simulink model "cc_main_multiple_points"  (R2016b)
settings: Solver=FixedStepAuto  StartTime=0.0  StopTime=inf  FixedStep=1e-3  RelTol=1e-3
values from neighbouring files (symbols this model uses):
  lx = 10    [multiple_points_platform_and_ball_characteristics.m]
  ly = 10    [multiple_points_platform_and_ball_characteristics.m]
libraries: MBDyn_collision_activator x3, MBDynCom x2
settings Model: Creator=matteo  LastModifiedBy=matteo

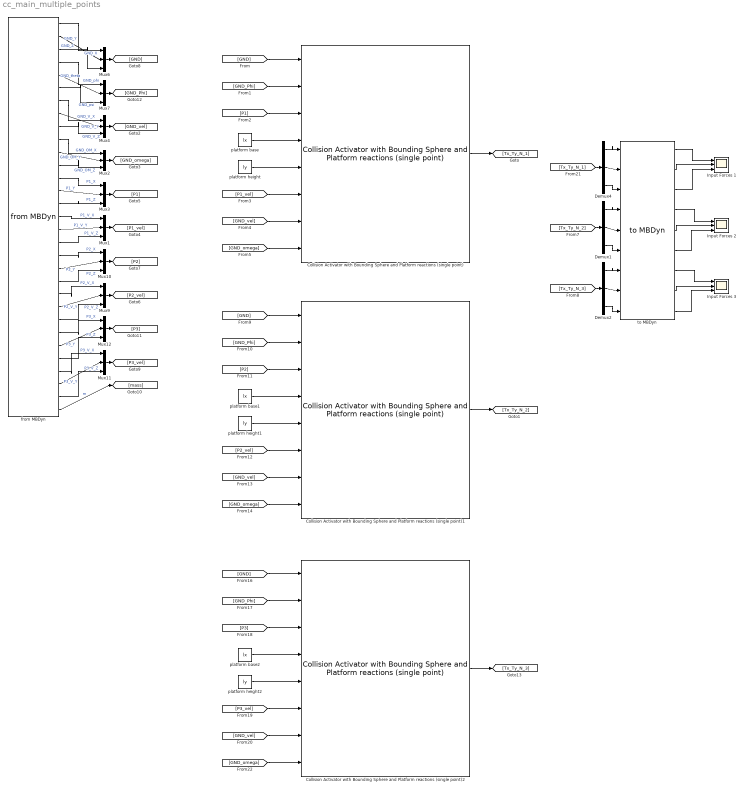
== system cc_main_multiple_points ==
  Collision Activator with Bounding Sphere and Platform reactions (single point) : MBDyn_collision_activator/Collision Activator with Bounding Sphere and Platform reactions (single point)  mult_factor=10  coulomb_friction_value=0  coefficient_viscous_friction=0.05  cosine_flag_threshold=3.9  local_distance_from_gnd_threshold=0  ground_stiffness=1e9  restitution_coeff=0.8  impact_speed_threshold=0.2  reaction_force_exponential=3  force_sign=-1  dissipation_coefficient_model=Flores
  Collision Activator with Bounding Sphere and Platform reactions (single point)1 : MBDyn_collision_activator/Collision Activator with Bounding Sphere and Platform reactions (single point)  mult_factor=10  coulomb_friction_value=0  coefficient_viscous_friction=0.05  cosine_flag_threshold=3.9  local_distance_from_gnd_threshold=0  ground_stiffness=1e9  restitution_coeff=0.8  impact_speed_threshold=0.2  reaction_force_exponential=3  force_sign=-1  dissipation_coefficient_model=Flores
  Collision Activator with Bounding Sphere and Platform reactions (single point)2 : MBDyn_collision_activator/Collision Activator with Bounding Sphere and Platform reactions (single point)  mult_factor=10  coulomb_friction_value=0  coefficient_viscous_friction=0.05  cosine_flag_threshold=3.9  local_distance_from_gnd_threshold=0  ground_stiffness=1e9  restitution_coeff=0.8  impact_speed_threshold=0.2  reaction_force_exponential=3  force_sign=-1  dissipation_coefficient_model=Flores
  Demux1 : Demux  Outputs=3
  Demux2 : Demux  Outputs=3
  Demux4 : Demux  Outputs=3
  Input Forces 1 : Scope  NumInputPorts=3
  Input Forces 2 : Scope  NumInputPorts=3
  Input Forces 3 : Scope  NumInputPorts=3
  Mux{1..4,6..7,9..12} (10 alike) : Mux  Inputs=3
  from MBDyn : MBDynCom/from MBDyn  Priority=0  RTAI_flag=off  Socket_flag=on  mbdtask='MBDTSK'  mbx='MBXINN'  net=on  node='127.0.0.1'  port=8001  path=''  N_chan=31  Tc=1.e-3
  platform base : Constant  Value=lx
  platform base1 : Constant  Value=lx
  platform base2 : Constant  Value=lx
  platform height : Constant  Value=ly
  platform height1 : Constant  Value=ly
  platform height2 : Constant  Value=ly
  to MBDyn : MBDynCom/to MBDyn  Priority=0  RTAI_flag=off  Socket_flag=on  mbdtask='MBDTSK'  mbx='MBXOUT'  net=on  node='127.0.0.1'  port=9001  path=''  N_chan=9  Tc=1e-3
  wires:
  to MBDyn/1 -> Input Forces 1/1
  from MBDyn/1 -> Mux6/1  "GND_X"
  from MBDyn/2 -> Mux6/2  "GND_Y"
  from MBDyn/4 -> Mux7/1  "GND_phi"
  from MBDyn/5 -> Mux7/2  "GND_theta"
  from MBDyn/6 -> Mux7/3  "GND_psi"
  from MBDyn/3 -> Mux6/3  "GND_Z"
  to MBDyn/2 -> Input Forces 1/2
  to MBDyn/3 -> Input Forces 1/3
  Mux7/1 -> [GND_Phi]
  Mux6/1 -> [GND]
  Demux4/1 -> to MBDyn/1
  Demux4/2 -> to MBDyn/2
  Demux4/3 -> to MBDyn/3
  [Tx_Ty_N_1] -> Demux4/1
  [GND] -> Collision Activator with Bounding Sphere and Platform reactions (single point)/1
  [GND_Phi] -> Collision Activator with Bounding Sphere and Platform reactions (single point)/2
  [P1] -> Collision Activator with Bounding Sphere and Platform reactions (single point)/3
  platform base/1 -> Collision Activator with Bounding Sphere and Platform reactions (single point)/4
  platform height/1 -> Collision Activator with Bounding Sphere and Platform reactions (single point)/5
  [GND_vel] -> Collision Activator with Bounding Sphere and Platform reactions (single point)/7
  [GND_omega] -> Collision Activator with Bounding Sphere and Platform reactions (single point)/8
  Collision Activator with Bounding Sphere and Platform reactions (single point)/1 -> [Tx_Ty_N_1]
  [P1_vel] -> Collision Activator with Bounding Sphere and Platform reactions (single point)/6
  Demux1/1 -> to MBDyn/4
  Demux1/2 -> to MBDyn/5
  Demux1/3 -> to MBDyn/6
  [Tx_Ty_N_2] -> Demux1/1
  Demux2/1 -> to MBDyn/7
  Demux2/2 -> to MBDyn/8
  Demux2/3 -> to MBDyn/9
  [Tx_Ty_N_3] -> Demux2/1
  to MBDyn/8 -> Input Forces 3/2
  to MBDyn/7 -> Input Forces 3/1
  to MBDyn/9 -> Input Forces 3/3
  to MBDyn/6 -> Input Forces 2/3
  to MBDyn/4 -> Input Forces 2/1
  to MBDyn/5 -> Input Forces 2/2
  from MBDyn/7 -> Mux4/1  "GND_V_X"
  from MBDyn/8 -> Mux4/2  "GND_V_Y"
  from MBDyn/9 -> Mux4/3  "GND_V_Z"
  from MBDyn/10 -> Mux2/1  "GND_OM_X"
  from MBDyn/11 -> Mux2/2  "GND_OM_Y"
  from MBDyn/12 -> Mux2/3  "GND_OM_Z"
  from MBDyn/31 -> [mass]  "m"
  Mux4/1 -> [GND_vel]
  Mux2/1 -> [GND_omega]
  from MBDyn/16 -> Mux1/1  "P1_V_X"
  from MBDyn/17 -> Mux1/2  "P1_V_Y"
  from MBDyn/18 -> Mux1/3  "P1_V_Z"
  Mux1/1 -> [P1_vel]
  from MBDyn/14 -> Mux3/2  "P1_Y"
  from MBDyn/13 -> Mux3/1  "P1_X"
  from MBDyn/15 -> Mux3/3  "P1_Z"
  Mux3/1 -> [P1]
  from MBDyn/22 -> Mux9/1  "P2_V_X"
  from MBDyn/23 -> Mux9/2  "P2_V_Y"
  from MBDyn/24 -> Mux9/3  "P2_V_Z"
  Mux9/1 -> [P2_vel]
  from MBDyn/20 -> Mux10/2  "P2_Y"
  from MBDyn/19 -> Mux10/1  "P2_X"
  from MBDyn/21 -> Mux10/3  "P2_Z"
  Mux10/1 -> [P2]
  from MBDyn/28 -> Mux11/1  "P3_V_X"
  from MBDyn/29 -> Mux11/2  "P3_V_Y"
  from MBDyn/30 -> Mux11/3  "P3_V_Z"
  Mux11/1 -> [P3_vel]
  from MBDyn/26 -> Mux12/2  "P3_Y"
  from MBDyn/25 -> Mux12/1  "P3_X"
  from MBDyn/27 -> Mux12/3  "P3_Z"
  Mux12/1 -> [P3]
  [GND] -> Collision Activator with Bounding Sphere and Platform reactions (single point)1/1
  [GND_Phi] -> Collision Activator with Bounding Sphere and Platform reactions (single point)1/2
  [P2] -> Collision Activator with Bounding Sphere and Platform reactions (single point)1/3
  platform base1/1 -> Collision Activator with Bounding Sphere and Platform reactions (single point)1/4
  platform height1/1 -> Collision Activator with Bounding Sphere and Platform reactions (single point)1/5
  [GND_vel] -> Collision Activator with Bounding Sphere and Platform reactions (single point)1/7
  [GND_omega] -> Collision Activator with Bounding Sphere and Platform reactions (single point)1/8
  Collision Activator with Bounding Sphere and Platform reactions (single point)1/1 -> [Tx_Ty_N_2]
  [P2_vel] -> Collision Activator with Bounding Sphere and Platform reactions (single point)1/6
  [GND] -> Collision Activator with Bounding Sphere and Platform reactions (single point)2/1
  [GND_Phi] -> Collision Activator with Bounding Sphere and Platform reactions (single point)2/2
  [P3] -> Collision Activator with Bounding Sphere and Platform reactions (single point)2/3
  platform base2/1 -> Collision Activator with Bounding Sphere and Platform reactions (single point)2/4
  platform height2/1 -> Collision Activator with Bounding Sphere and Platform reactions (single point)2/5
  [GND_vel] -> Collision Activator with Bounding Sphere and Platform reactions (single point)2/7
  [GND_omega] -> Collision Activator with Bounding Sphere and Platform reactions (single point)2/8
  Collision Activator with Bounding Sphere and Platform reactions (single point)2/1 -> [Tx_Ty_N_3]
  [P3_vel] -> Collision Activator with Bounding Sphere and Platform reactions (single point)2/6
